simulink model "NovoModeloControlePorPressaoRev2_Resist"  (R2017a)
settings: Solver=ode3  StartTime=0.0  StopTime=Tsimulacao  FixedStep=Tamostra  RelTol=1e-3  EnableMultiTasking=on
values from neighbouring files (symbols this model uses):
  Delay = 0.01    [CodigoTeste.m]    (also in CodigoTesteSimulador.m = 1.5; ControlePorPressaoRevFinal.m = input('Escolha o tempo para o delay do ventilador [s] '); PlotsDaSimulacaoFinal.m = 0.05; SimulacaoFinalDaPesquisa.m = ResultadosVentiladorInterrupcaoIntermitente(i,6))
  E = 38.1970    (= 38.197)    [CodigoTeste.m]    (also in CodigoTesteSimulador.m; ControlePorPressaoRevFinal.m = 50; PlotsDaSimulacaoFinal.m = 8.33333333333; SimulacaoFinalDaPesquisa.m = 1/ResultadosVentiladorInterrupcaoIntermitente(i,5))
  Limite_Vazao = 0.5    [CodigoTeste.m]    (also in ControlePorPressaoRevFinal.m = input('Escolha a vazão máxima entregue pelo o ventilador [L/; PlotsDaSimulacaoFinal.m; SimulacaoFinalDaPesquisa.m; Untitled.m = 1)
  PaspMax = Pasp(1,3)    [CodigoTeste.m]    (also in CodigoTesteSimulador.m; Untitled.m = 3)
  PaspMed = Pasp(1,2)    [CodigoTeste.m]    (also in CodigoTesteSimulador.m; Untitled.m = 2)
  PaspMin = Pasp(1,1)    [CodigoTeste.m]    (also in CodigoTesteSimulador.m; Untitled.m = 1)
  PressaoDelay = Pvent    (= 5)    [CodigoTeste.m]    (also in CodigoTesteSimulador.m; ControlePorPressaoRevFinal.m = 10; PlotsDaSimulacaoFinal.m = 10; SimulacaoFinalDaPesquisa.m = 10)
  Ptrigger = 0.0    (= 0)    [CodigoTeste.m]    (also in CodigoTesteSimulador.m = 0.5; ControlePorPressaoRevFinal.m = input('Escolha a pressão de trigger do ventilador [cmH2O] '); PlotsDaSimulacaoFinal.m = 0.5; SimulacaoFinalDaPesquisa.m = ResultadosVentiladorInterrupcaoIntermitente(i,7))
  Pvent = 5    [CodigoTeste.m]    (also in CodigoTesteSimulador.m; ControlePorPressaoRevFinal.m = 10; PlotsDaSimulacaoFinal.m = 10; SimulacaoFinalDaPesquisa.m = 10)
  Rrs = 3.3464    [CodigoTeste.m]    (also in CodigoTesteSimulador.m; ControlePorPressaoRevFinal.m = 5; PlotsDaSimulacaoFinal.m = 5; SimulacaoFinalDaPesquisa.m = ResultadosVentiladorInterrupcaoIntermitente(i,4))
  Tamanho_Sonda = 10    [CodigoTeste.m]    (also in CodigoTesteSimulador.m; ControlePorPressaoRevFinal.m = input('Qual o tamanho da sonda utilizada [FR]? 00, 06, 08, 1; PlotsDaSimulacaoFinal.m = 6; SimulacaoFinalDaPesquisa.m = ResultadosVentiladorInterrupcaoIntermitente(i,9))
  TOT = 7.5    [CodigoTeste.m]    (also in CodigoTesteSimulador.m; ControlePorPressaoRevFinal.m = input('Qual o tamanho do Tubo Orotraquial utilizado [mm]? 7.; PlotsDaSimulacaoFinal.m; SimulacaoFinalDaPesquisa.m = ResultadosVentiladorInterrupcaoIntermitente(i,8))
  VolumeInicial = VR+PressaoInicial/E    (= 0.130900332487)    [CodigoTeste.m]    (also in CodigoTesteSimulador.m; ControlePorPressaoRevFinal.m = 1.4; PlotsDaSimulacaoFinal.m = 2.4; SimulacaoFinalDaPesquisa.m = 2.4)
  VR = 0    [CodigoTeste.m]    (also in CodigoTesteSimulador.m; ControlePorPressaoRevFinal.m = 1.2; PlotsDaSimulacaoFinal.m = 1.2; SimulacaoFinalDaPesquisa.m = 1.2)
libraries: simulink x1
settings Model: Creator=Proprietário  LastModifiedBy=Texugão
settings DataIOCC: LimitDataPoints=on  SaveFormat=Array
settings OptimizationCC: LifeSpan=inf
settings DebuggingCC: SolverPrmCheckMsg=warning  SFUnexpectedBacktrackingDiag=warning  SFNoUnconditionalDefaultTransitionDiag=warning  SFExecutionAtInitializationDiag=none
settings HardwareCC: ProdBitPerPointer=32  ProdBitPerSizeT=32  ProdBitPerPtrDiffT=32  ProdLargestAtomicFloat=None  ProdIntDivRoundTo=Undefined  ProdEndianess=Unspecified  ProdWordSize=32  ProdHWDeviceType=32-bit Generic
settings ModelReferenceCC: PropagateSignalLabelsOutOfModel=off
settings GRTTargetCC: TargetLangStandard=C89/C90 (ANSI)  GeneratePreprocessorConditionals=Disable all
settings ConfigComp: CovMetricSettings=dw  CovHtmlReporting=on  CovSaveCumulativeToWorkspaceVar=on  CovSaveSingleToWorkspaceVar=on  CovExternalEMLEnable=off  CovSFcnEnable=off

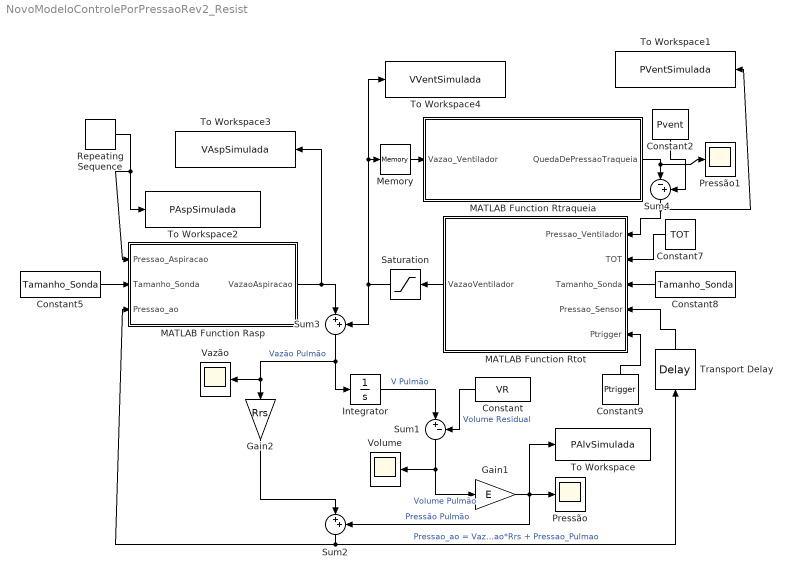
== system NovoModeloControlePorPressaoRev2_Resist ==
  Constant : Constant  Value=VR
  Constant2 : Constant  Value=Pvent
  Constant5 : Constant  Value=Tamanho_Sonda
  Constant7 : Constant  Value=TOT
  Constant8 : Constant  Value=Tamanho_Sonda
  Constant9 : Constant  Value=Ptrigger
  Gain1 : Gain  Gain=E
  Gain2 : Gain  Gain=Rrs
  Integrator : Integrator  InitialCondition=VolumeInicial
  MATLAB Function Rasp : MATLAB Function  TreatAsAtomicUnit=on
  MATLAB Function Rtot : MATLAB Function  TreatAsAtomicUnit=on
  MATLAB Function Rtraqueia : MATLAB Function  TreatAsAtomicUnit=on
  Memory : Memory
  Pressão : Scope
  Pressão1 : Scope
  Repeating Sequence : simulink/Sources/Repeating Sequence  rep_seq_t=[0 5 5+0.001 20 20+0.001 40 40+0.001 55 55+0.001 75 75+0.001 90 90+0.001 95]  rep_seq_y=[0 0 PaspMin PaspMin 0 0 PaspMed PaspMed 0 0 PaspMax PaspMax 0 0]
  Saturation : Saturate  UpperLimit=Limite_Vazao  LowerLimit=-Limite_Vazao
  Sum1 : Sum  Inputs=|+-
  Sum2 : Sum  Inputs=|++
  Sum3 : Sum  Inputs=|++
  Sum4 : Sum  Inputs=|-+
  To Workspace : ToWorkspace  VariableName=PAlvSimulada  SaveFormat=Timeseries  SampleTime=-1
  To Workspace1 : ToWorkspace  VariableName=PVentSimulada  SaveFormat=Timeseries  SampleTime=-1
  To Workspace2 : ToWorkspace  VariableName=PAspSimulada  SaveFormat=Timeseries  SampleTime=-1
  To Workspace3 : ToWorkspace  VariableName=VAspSimulada  SaveFormat=Timeseries  SampleTime=-1
  To Workspace4 : ToWorkspace  VariableName=VVentSimulada  SaveFormat=Timeseries  SampleTime=-1
  Transport Delay : TransportDelay  DelayTime=Delay  InitialOutput=PressaoDelay
  Vazão : Scope
  Volume : Scope
  wires:
  Integrator/1 -> Sum1/1  "V Pulmão"
  Constant/1 -> Sum1/2  "Volume Residual"
  Sum3/1 -> Integrator/1, Vazão/1, Gain2/1  "Vazão Pulmão"
  Sum1/1 -> Gain1/1, Volume/1  "Volume Pulmão"
  Constant5/1 -> MATLAB Function Rasp/2(Tamanho_Sonda)
  Constant8/1 -> MATLAB Function Rtot/3(Tamanho_Sonda)
  Constant7/1 -> MATLAB Function Rtot/2(TOT)
  Transport Delay/1 -> MATLAB Function Rtot/4(Pressao_Sensor)
  Constant9/1 -> MATLAB Function Rtot/5(Ptrigger)
  MATLAB Function Rasp/1(VazaoAspiracao) -> To Workspace3/1, Sum3/1
  Gain1/1 -> To Workspace/1, Pressão/1, Sum2/2  "Pressão Pulmão"
  Gain2/1 -> Sum2/1
  Sum2/1 -> MATLAB Function Rasp/3(Pressao_ao), Transport Delay/1  "Pressao_ao = Vazao_Pulmao*Rrs + Pressao_Pulmao"
  MATLAB Function Rtot/1(VazaoVentilador) -> Saturation/1
  Saturation/1 -> Memory/1, To Workspace4/1, Sum3/2
  Repeating Sequence/1 -> MATLAB Function Rasp/1(Pressao_Aspiracao), To Workspace2/1
  Constant2/1 -> Sum4/2
  Sum4/1 -> To Workspace1/1, MATLAB Function Rtot/1(Pressao_Ventilador)
  MATLAB Function Rtraqueia/1(QuedaDePressaoTraqueia) -> Pressão1/1, Sum4/1
  Memory/1 -> MATLAB Function Rtraqueia/1(Vazao_Ventilador)

== matlab function NovoModeloControlePorPressaoRev2_Resist/MATLAB Function Rtraqueia ==
  data: Vazao_Ventilador input; QuedaDePressaoTraqueia output
function QuedaDePressaoTraqueia = ResistenciaTraqueia(Vazao_Ventilador)

% QuedaDePressaoTraqueia = 81.53 * Vazao_Ventilador^2 + 13.93 * Vazao_Ventilador;
QuedaDePressaoTraqueia = 20.97 * Vazao_Ventilador;

end

== matlab function NovoModeloControlePorPressaoRev2_Resist/MATLAB Function Rasp ==
  data: Pressao_Aspiracao input; Tamanho_Sonda input; Pressao_ao input; VazaoAspiracao output
function VazaoAspiracao = VazaoAspiracao(Pressao_Aspiracao, Tamanho_Sonda, Pressao_ao)

%Bug do Simulink está tratando os sinais como complexos. 
%Então se trabalha com o modulo
Delta_P = abs(Pressao_Aspiracao - Pressao_ao);

%Correção do sinal pelo o Bug
Sinal = 1;
if Pressao_Aspiracao < Pressao_ao
    %Pressão Aspiração mais negativa que o paciente
    Sinal = -1;
else
    %Pressão do paciente mais negativa que a pressão Aspiração
    %Aspiração não entrega fluxo no sentido contrario
    Sinal = 1;
end

%Estimação da Vazão de acordo com o Tamanho da Sonda utilizada [00, 06, 08, 10, ou 12]
Vazao = 1;
Rasp = 1;
if Tamanho_Sonda == 0
    Vazao = 0;
elseif Tamanho_Sonda == 06
    Vazao = 0.001339*Delta_P^0.7939;   
elseif Tamanho_Sonda == 08
    Vazao = 0.01081*Delta_P^0.6338;
elseif Tamanho_Sonda == 10
    Vazao = 0.01501*Delta_P^0.6046;
elseif Tamanho_Sonda == 12
    Vazao = 0.03048*Delta_P^0.5689;
elseif Tamanho_Sonda == 14
    Vazao = 0.05087*Delta_P^0.5644;
end

VazaoAspiracao = Sinal*Vazao;

end

== matlab function NovoModeloControlePorPressaoRev2_Resist/MATLAB Function Rtot ==
  data: Pressao_Ventilador input; TOT input; Tamanho_Sonda input; Pressao_Sensor input; VazaoVentilador output; Ptrigger input
function VazaoVentilador = VazaoVentilador(Pressao_Ventilador, TOT, Tamanho_Sonda, Pressao_Sensor, Ptrigger)

%Bug do Simulink está tratando os sinais como complexos. 
%Então se trabalha com o modulo
Delta_P = abs(Pressao_Ventilador - Pressao_Sensor);

%Correção do sinal pelo o Bug
Sinal = 1;
if Pressao_Ventilador < Pressao_Sensor
    %Pressao do ventilador menor que a pressão do paciente
    %Apenas desliga o ventilador
    Sinal = -1;
else
    Sinal = 1;
end

%Sensibilidade do Ventilador
persistent Status_Ventilador; %A variável Status_Ventilador mantem o valor entre execuções
if isempty(Status_Ventilador)
    %Se está vazio, começa desligado
    Status_Ventilador=false;
end
if Delta_P == 0     
    %Desliga o Ventilador
    Status_Ventilador = false;
elseif Delta_P > Ptrigger
    %Ativa o ventilador
    Status_Ventilador = true;
end

if Status_Ventilador
    %Mantem o Delta_P
else
    %Se o ventilador desligado, não tem vazão
    Delta_P =0;
end 

%Estimação da Vazão de acordo com a combinação de TOT [7.5 ou 8.5] e Tamanho da Sonda utilizada [00, 06, 08, 10, ou 12]
Vazao = 1;
Rtot = 1;
if TOT == 7.5
    if Tamanho_Sonda == 0
        Vazao = 0.3833*Delta_P^0.5872;
    elseif Tamanho_Sonda == 06
        Vazao = 0.3223*Delta_P^0.5745;
    elseif Tamanho_Sonda == 08
        Vazao = 0.2745*Delta_P^0.5687;
    elseif Tamanho_Sonda == 10
        Vazao = 0.2682*Delta_P^0.5726;
    end
elseif TOT == 8.5
    if Tamanho_Sonda == 0
        Vazao = 0.548*Delta_P^0.5688;
    elseif Tamanho_Sonda == 06
        Vazao = 0.4413*Delta_P^0.5807;
    elseif Tamanho_Sonda == 08
        Vazao = 0.3795*Delta_P^0.5819;
    elseif Tamanho_Sonda == 10
        Vazao = 0.3808*Delta_P^0.5843;
    elseif Tamanho_Sonda == 12
        Vazao = 0.321*Delta_P^0.5871;
    end
end

% if Vazao > 0.5 %Vazão máxima do ventilador
%     Vazao = 0.5;
% end

VazaoVentilador = Sinal*Vazao;

end
